simulink model "NTCM_Procedure"  (R2021a)
settings: Solver=FixedStepAuto  StartTime=0.0  StopTime=End_Time  FixedStep=Sample_Time  RelTol=1e-3  EnableMultiTasking=on
model workspace (MAT data in the model file):
  ErrCodeEl = Simulink.Parameter
  ErrCodeEl.Value = 1
  ErrCodeEl.DataType = 'uint16'
  ErrCodeEl.Dimensions = [1 1]
  ErrCodeIn = Simulink.Parameter
  ErrCodeIn.Value = 1
  ErrCodeIn.DataType = 'uint16'
  ErrCodeIn.Dimensions = [1 1]
  ErrCodeOut = Simulink.Parameter
  ErrCodeOut.Value = 1
  ErrCodeOut.DataType = 'uint16'
  ErrCodeOut.Dimensions = [1 1]
  ErrVarCheckIn = Simulink.Parameter
  ErrVarCheckIn.Value = [0; 0; 0; 0; 0; 0; 0; 0; 0; 0; 0; 0]
  ErrVarCheckIn.DataType = 'auto'
  ErrVarCheckIn.Dimensions = [12 1]
  ErrVarCheckOut = Simulink.Parameter
  ErrVarCheckOut.Value = [0; 0; 0]
  ErrVarCheckOut.DataType = 'auto'
  ErrVarCheckOut.Dimensions = [3 1]
  ErrVarEl = Simulink.Parameter
  ErrVarEl.Value = 0
  ErrVarEl.DataType = 'auto'
  ErrVarEl.Dimensions = [1 1]
  IPP_RefAltitude = Simulink.Parameter
  IPP_RefAltitude.Value = 450000
  IPP_RefAltitude.DataType = 'auto'
  IPP_RefAltitude.Dimensions = [1 1]
  LTd = Simulink.Parameter
  LTd.Value = 14
  LTd.DataType = 'auto'
  LTd.Dimensions = [1 1]
  NoErr = Simulink.Parameter
  NoErr.Value = 0
  NoErr.DataType = 'uint16'
  NoErr.Dimensions = [1 1]
  Pf1 = Simulink.Parameter
  Pf1.Value = 0.4
  Pf1.DataType = 'auto'
  Pf1.Dimensions = [1 1]
  RangeLwEl = Simulink.Parameter
  RangeLwEl.Value = 0
  RangeLwEl.DataType = 'auto'
  RangeLwEl.Dimensions = [1 1]
  RangeLwIn = Simulink.Parameter
  RangeLwIn.Value = [0; -4; -0.25; 1; 0; -90; -180; -4000; -90; -180; 450000; 0]
  RangeLwIn.DataType = 'auto'
  RangeLwIn.Dimensions = [12 1]
  RangeLwOut = Simulink.Parameter
  RangeLwOut.Value = [0; 0; 0]
  RangeLwOut.DataType = 'auto'
  RangeLwOut.Dimensions = [3 1]
  RangeUpEl = Simulink.Parameter
  RangeUpEl.Value = 1.57079632679
  RangeUpEl.DataType = 'auto'
  RangeUpEl.Dimensions = [1 1]
  RangeUpIn = Simulink.Parameter
  RangeUpIn.Value = [512; 4; 0.25; 366; 24; 90; 180; 400000; 90; 180; 600000000; 20000000000]
  RangeUpIn.DataType = 'auto'
  RangeUpIn.Dimensions = [12 1]
  RangeUpOut = Simulink.Parameter
  RangeUpOut.Value = [500; 1500; 1000000000000]
  RangeUpOut.DataType = 'auto'
  RangeUpOut.Dimensions = [3 1]
  Re = Simulink.Parameter
  Re.Value = 6371000
  Re.DataType = 'auto'
  Re.Dimensions = [1 1]
  doy_DAV = Simulink.Parameter
  doy_DAV.Value = 18
  doy_DAV.DataType = 'auto'
  doy_DAV.Dimensions = [1 1]
  doy_DSAV = Simulink.Parameter
  doy_DSAV.Value = 6
  doy_DSAV.DataType = 'auto'
  doy_DSAV.Dimensions = [1 1]
  k1 = Simulink.Parameter
  k1.Value = 0.92519
  k1.DataType = 'auto'
  k1.Dimensions = [1 1]
  k10 = Simulink.Parameter
  k10.Value = 1.20556
  k10.DataType = 'auto'
  k10.Dimensions = [1 1]
  k11 = Simulink.Parameter
  k11.Value = 1.41808
  k11.DataType = 'auto'
  k11.Dimensions = [1 1]
  k12 = Simulink.Parameter
  k12.Value = 0.13985
  k12.DataType = 'auto'
  k12.Dimensions = [1 1]
  k2 = Simulink.Parameter
  k2.Value = 0.16951
  k2.DataType = 'auto'
  k2.Dimensions = [1 1]
  k3 = Simulink.Parameter
  k3.Value = 0.00443
  k3.DataType = 'auto'
  k3.Dimensions = [1 1]
  k4 = Simulink.Parameter
  k4.Value = 0.06626
  k4.DataType = 'auto'
  k4.Dimensions = [1 1]
  k5 = Simulink.Parameter
  k5.Value = 0.00899
  k5.DataType = 'auto'
  k5.Dimensions = [1 1]
  k6 = Simulink.Parameter
  k6.Value = 0.21289
  k6.DataType = 'auto'
  k6.Dimensions = [1 1]
  k7 = Simulink.Parameter
  k7.Value = -0.15414
  k7.DataType = 'auto'
  k7.Dimensions = [1 1]
  k8 = Simulink.Parameter
  k8.Value = -0.38439
  k8.DataType = 'auto'
  k8.Dimensions = [1 1]
  k9 = Simulink.Parameter
  k9.Value = 1.14023
  k9.DataType = 'auto'
  k9.Dimensions = [1 1]
  lamGNP_deg = Simulink.Parameter
  lamGNP_deg.Value = -71.78
  lamGNP_deg.DataType = 'auto'
  lamGNP_deg.Dimensions = [1 1]
  phiGNP_deg = Simulink.Parameter
  phiGNP_deg.Value = 79.74
  phiGNP_deg.DataType = 'auto'
  phiGNP_deg.Dimensions = [1 1]
  phi_c1 = Simulink.Parameter
  phi_c1.Value = 16
  phi_c1.DataType = 'auto'
  phi_c1.Dimensions = [1 1]
  phi_c2 = Simulink.Parameter
  phi_c2.Value = -10
  phi_c2.DataType = 'auto'
  phi_c2.Dimensions = [1 1]
  sigma_c1 = Simulink.Parameter
  sigma_c1.Value = 12
  sigma_c1.DataType = 'auto'
  sigma_c1.Dimensions = [1 1]
  sigma_c2 = Simulink.Parameter
  sigma_c2.Value = 13
  sigma_c2.DataType = 'auto'
  sigma_c2.Dimensions = [1 1]
Description:
  | Model NTCM Procedure
settings Model: ModifiedByFormat=Francesco Menzione  OrderedModelArguments=off  Creator=Francesco Menzione  LastModifiedBy=Francesco Menzione
settings DataIOCC: ReturnWorkspaceOutputs=off  SignalLoggingName=logsout_new
settings OptimizationCC: UseDivisionForNetSlopeComputation=on  UseFloatMulNetSlope=on  UseSpecifiedMinMax=on  BufferReuse=off  PassReuseOutputArgsAs=Individual arguments  ZeroExternalMemoryAtStartup=off  ZeroInternalMemoryAtStartup=off  EfficientFloat2IntCast=on  LifeSpan=2  EfficientTunableParamExpr=on
settings DebuggingCC: ParameterTunabilityLossMsg=error  AssertControl=DisableAll  SFMachineParentedDataDiag=warning
settings HardwareCC: ProdBitPerPointer=32  ProdBitPerSizeT=32  ProdBitPerPtrDiffT=32  ProdLargestAtomicInteger=LongLong  ProdLargestAtomicFloat=Double  ProdEndianess=BigEndian  ProdWordSize=32  ProdLongLongMode=on  ProdHWDeviceType=Custom Processor->Custom
settings SFSimCC: MATLABDynamicMemAlloc=off
settings RTWCC: SystemTargetFile=ert.tlc  TemplateMakefile=ert_default_tmf  GenerateReport=on  CustomDefine=CheckOn=1  Toolchain=MinGW64 | gmake (64-bit Windows)  BuildConfiguration=Faster Runs  LaunchReport=on  PortableWordSizes=on  CodeExecutionProfiling=on  CodeProfilingInstrumentation=detailed  GenerateTraceReportSl=on  GenerateTraceReportSf=on  GenerateTraceReportEml=on  GenerateWebview=on  GenerateCodeMetricsReport=on  CheckMdlBeforeBuild=Warning
settings CodeAppCC: IgnoreCustomStorageClasses=off  OperatorAnnotations=on  SimulinkDataObjDesc=on  CustomSymbolStrFcn=$M$F  CustomSymbolStrFcnArg=$N$M  CustomSymbolStrBlkIO=lOut_$N$M  InsertBlockDesc=on  SimulinkBlockComments=off
settings ERTTargetCC: TargetLangStandard=C99 (ISO)  UtilityFuncGeneration=Shared location  GenerateSampleERTMain=on  CombineSignalStateStructs=on  SuppressErrorStatus=on  CodeInterfacePackaging=Reusable function  SupportNonFinite=off  SupportComplex=off  RemoveResetFunc=off  ParenthesesLevel=Maximum  CastingMode=Standards  RootIOFormat=Structure reference  ERTSrcFileBannerTemplate=JRCert_code_template.cgt  ERTHdrFileBannerTemplate=JRCert_code_template.cgt  ERTDataSrcFileTemplate=JRCert_code_template.cgt  ERTDataHdrFileTemplate=JRCert_code_template.cgt  ERTCustomFileTemplate=example_file_process.tlc  EnableSignedLeftShifts=off  EnableSignedRightShifts=off

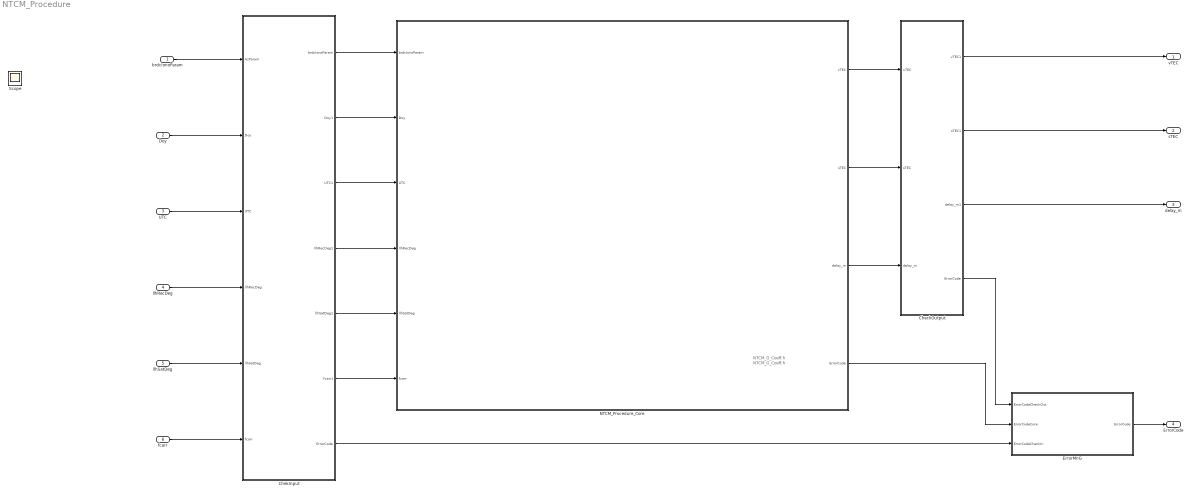
== system NTCM_Procedure ==
  note: NTCM_G_Coeff.h
  note: NTCM_G_Coeff.h
  brdcIonoParam : Inport  PortDimensions=[3,1]
  Doy : Inport  Port=2  PortDimensions=1
  UTC : Inport  Port=3  PortDimensions=1
  llhRecDeg : Inport  Description=dxdxxdxhx  Port=4  PortDimensions=[3,1]
  llhSatDeg : Inport  Port=5  PortDimensions=[3,1]
  fcarr : Inport  Port=6  PortDimensions=1
  CheckOutput : Subsystem  Description=|  TreatAsAtomicUnit=on  RTWFcnName=CheckOutput
      | FUNCTION:
      |    ------
      |    The function check that all output lie within the expected range and perform
      |    correspondent saturation when needed
      |    
      |    INPUT:
      |    ------
      | /n vTEC => Vertical TEC [TECU]
      | /n sTEC => Slant TEC [TECU]
      | /n delay_m=> Ionospheric Delay [m]
      | /n llhRecDeg => User position in Longitude[rad], Latitude[rad], height[m] 
      | /n llhSatDeg => Satellite position in Longitude[rad], Latitude[rad], height[m]  
      | /n fcarr => Carrier frequency
      |    
      |    OUTPUT:
      |    ------
      | /n lOutCheck_Input => Validated  Output vector [1,2,3]
      | /n lOut_ErrorCheckIn =>Validity  Output flag [1,2,3]
      settings: RTWFcnNameOpts=User specified  RTWFileNameOpts=Use function name
  ChekInput : Subsystem  Description=|  TreatAsAtomicUnit=on  RTWFcnName=ChekInput
      | FUNCTION:
      |    ------
      |    The function check that all input lie within the expected range and perform
      |    correspondent saturation when needed
      |    
      |    INPUT:
      |    ------
      |    AzPara => Az0, Az1 and Az2 Iono Parameters broadcasted by Galileo
      | \n Doy => Day of the year 
      | \n UTC => UTC Time in hours (0 for midnight)
      | \n llhRecDeg => User position in Longitude[rad], Latitude[rad], height[m] 
      | \n llhSatDeg => Satellite position in Longitude[rad], Latitude[rad], height[m]  
      | \n fcarr => Carrier frequency
      |    
      |    OUTPUT:
      | -  -----
      |    lOutCheck_Input => Validated Input vector [1,...12]
      | \n lOut_ErrorCheckIn =>Validity Flags [1,...12]
      settings: RTWFcnNameOpts=User specified  RTWFileNameOpts=Use function name
  ErrorMnG : Subsystem  Description=|  TreatAsAtomicUnit=on  RTWFcnName=ErrorMnG
      | ChekOutput
      |    FUNCTION:
      |    ------
      |    The function ccollect all errors log in a unique vector of unsigned integers
      |    
      |    INPUT:
      |    ------
      |    ErrorCodeCheckOut => Error Code for Output Interface 
      | /n ErrorCodeCore => Error Code for Core 
      | /n ErrorCodeCheckIn =>Error Code for Input  Interface 
      |    
      |    OUTPUT:
      |    ------
      | /n ErrorCode =>Final Err Code Vector [ ErrorCodeCheckOut,ErrorCodeCore,ErrorCodeCheckIn
      settings: RTWFcnNameOpts=User specified  RTWFileNameOpts=Use function name
  NTCM_Procedure_Core : Subsystem  Description=|  TreatAsAtomicUnit=on  RTWFcnName=NTCM_Procedure_Core
      | <strong> FUNCTION </strong>
      |     The core function implements the step-by-step procedure as described in [1].
      |    The "core" suffix aim at sparating this pure algorithmic block from any consistency/control
      |    or I/O logic implemented externally by the user ( the check-in/checkout steps included in the
      |    overall procedure are provided just an example of possible wrapping. It is worthy to remind
      |    that in order to implement the ionospheric algorithm for Galileo single frequency receivers
      |    for each satellite-user line-of-sight the following steps shall be followed:
      |    \n 1) Obtain estimates of user receiver position (lat,long,h)_i, satellite position (lat,long,h)_j
      |    \n 2) Universal Time (UT), in terms of time of day and month
      |    \n 3) Obtain Effective Ionisation Level Azpar and broadcast coefficients (a_i0,a_i1,a_i2 )
      |    \n 4)Calculate satellite elevation (E) and azimuth (A) angles
      |    \n 5)Calculate ionospheric pierce point location for the user-to-satellite
      |    \n 6) Call NTCM_G to calculate VTEC at pierce point location and local time (LT)
      |    \n   (Section 2.5.4 in[1] provides a formula to convert UT to LT).
      |    \n 7) Calculate ionospheric Mapping Function (MF) using the equation provided in Section 2.5.8.
      |    \n 8) Convert VTEC to STEC using the ionospheric mapping function.
      |    \n 9) Convert STEC to time delay using Eq. 1 in[1] for the corresponding frequency to obtain
      |    \n the correction
      |    \n 10) Apply correction to selected link
      | 
      |    @param[in] AzPara  		=> alpha0, alpha1, and alpha2 Iono Parameters broadcasted by Galileo
      |    @param[in] Doy  		=> Day of the year
      |    @param[in] UTC   		=> UTC Time in hours (0 for midnight)
      |    @param[in] llhRecDeg   		=> User position in Longitude[rad], Latitude[rad], height[m]
      |    @param[in] llhSatDeg  		=> Satellite position in Longitude[rad], Latitude[rad], height[m]
      |    @param[in] fcarr  		=> Carrier frequency
      | 
      |    @param[out] vTEC  		=> Vertical TEC
      |    @param[out] sTEC  		=> Slant TEC
      |    @param[out] delay_m  		=> Signal propagation time delay in [m]
      |    @param[out] ErrorCode  		=> Error Code (optional)
      | 
      |  
      |  <strong> Tuning Constant </strong>
      |   <table>
      |  <tr><th> Label                      <th>Value       
      |  <tr><td> ErrCodeEl <td> 2U 
      |  <tr><td> ErrCodeEl  		<td>2U                        
      |  <tr><td> ErrCodeIn  		<td>1U
      |  <tr><td> ErrCodeOut  	<td>3U
      |  <tr><td> IPP_RefAltitude <td> 450000.0                  
      |  <tr><td> LTd  			<td>14.0
      |  <tr><td> NoErr  			<td>0U
      |  <tr><td> Pf1  			<td>0.4
      |  <tr><td> doy_DAV  		<td>18.0
      |  <tr><td> doy_DSAV  		<td>6.0
      |  <tr><td> lamGNP_deg  	<td>-71.78
      |  <tr><td> phiGNP_deg  	<td>79.74
      |  <tr><td> phi_c1  		<td>16.0
      |  <tr><td> phi_c2  		<td>-10.0
      |  <tr><td> sigma_c1  		<td>12.0
      |  <tr><td> sigma_c2  		<td>13.0
      |  <tr><td> k1  			<td>0.92519
      |  <tr><td> k10  			<td>1.20556
      |  <tr><td> k11  			<td>1.41808
      |  <tr><td> k12  			<td>0.13985
      |  <tr><td> k2  			<td>0.16951
      |  <tr><td> k3  			<td>0.00443
      |  <tr><td> k4  			<td>0.06626
      |  <tr><td> k5  			<td>0.00899
      |  <tr><td> k6  			<td>0.21289
      |  <tr><td> k7  			<td>-0.15414
      |  <tr><td> k8  			<td>-0.38439
      |  <tr><td> k9  			<td>1.14023
      | </table>
      | @ingroup NTCM_Procedure
      | @file
      settings: RTWFcnNameOpts=User specified  RTWFileNameOpts=Use function name
  vTEC : Outport
  sTEC : Outport  Port=2
  delay_m : Outport  Port=3
  ErrorCode : Outport  Port=4
  Scope : Scope
  wires:
  CheckOutput/1(vTEC1) -> vTEC/1
  CheckOutput/2(sTEC1) -> sTEC/1
  ErrorMnG/1(ErrorCode) -> ErrorCode/1
  CheckOutput/3(delay_m1) -> delay_m/1
  brdcIonoParam/1 -> ChekInput/1(AzParam)
  Doy/1 -> ChekInput/2(Doy)
  UTC/1 -> ChekInput/3(UTC)
  llhRecDeg/1 -> ChekInput/4(llhRecDeg)
  llhSatDeg/1 -> ChekInput/5(llhSatDeg)
  fcarr/1 -> ChekInput/6(fcarr)
  ChekInput/1(brdcIonoParam) -> NTCM_Procedure_Core/1(brdcIonoParam)
  ChekInput/2(Doy1) -> NTCM_Procedure_Core/2(Doy)
  ChekInput/3(UTC1) -> NTCM_Procedure_Core/3(UTC)
  ChekInput/4(llhRecDeg1) -> NTCM_Procedure_Core/4(llhRecDeg)
  ChekInput/5(llhSatDeg1) -> NTCM_Procedure_Core/5(llhSatDeg)
  ChekInput/6(fcarr1) -> NTCM_Procedure_Core/6(fcarr)
  NTCM_Procedure_Core/1(vTEC) -> CheckOutput/1(vTEC)
  NTCM_Procedure_Core/2(sTEC) -> CheckOutput/2(sTEC)
  NTCM_Procedure_Core/3(delay_m) -> CheckOutput/3(delay_m)
  CheckOutput/4(ErrorCode) -> ErrorMnG/1(ErrorCodeCheckOut)
  NTCM_Procedure_Core/4(ErrorCode) -> ErrorMnG/2(ErrorCodeCore)
  ChekInput/7(ErrorCode) -> ErrorMnG/3(ErrorCodeCheckIn)

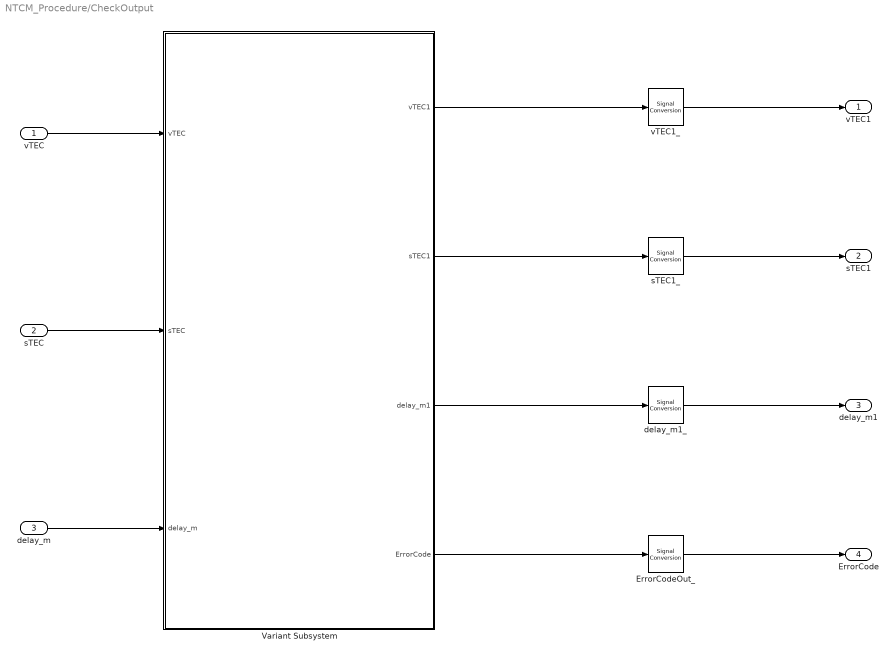
== system NTCM_Procedure/CheckOutput ==
  vTEC : Inport
  sTEC : Inport  Port=2
  delay_m : Inport  Port=3
  ErrorCodeOut_ : SignalConversion  OverrideOpt=off
  Variant Subsystem : Subsystem  Variant=on  VariantActivationTime=code compile
  delay_m1_ : SignalConversion  OverrideOpt=off
  sTEC1_ : SignalConversion  OverrideOpt=off
  vTEC1_ : SignalConversion  OverrideOpt=off
  vTEC1 : Outport
  sTEC1 : Outport  Port=2
  delay_m1 : Outport  Port=3
  ErrorCode : Outport  Port=4
  wires:
  Variant Subsystem/2(sTEC1) -> sTEC1_/1
  delay_m/1 -> Variant Subsystem/3(delay_m)
  vTEC/1 -> Variant Subsystem/1(vTEC)
  Variant Subsystem/1(vTEC1) -> vTEC1_/1
  Variant Subsystem/3(delay_m1) -> delay_m1_/1
  Variant Subsystem/4(ErrorCode) -> ErrorCodeOut_/1
  sTEC/1 -> Variant Subsystem/2(sTEC)
  vTEC1_/1 -> vTEC1/1
  sTEC1_/1 -> sTEC1/1
  delay_m1_/1 -> delay_m1/1
  ErrorCodeOut_/1 -> ErrorCode/1

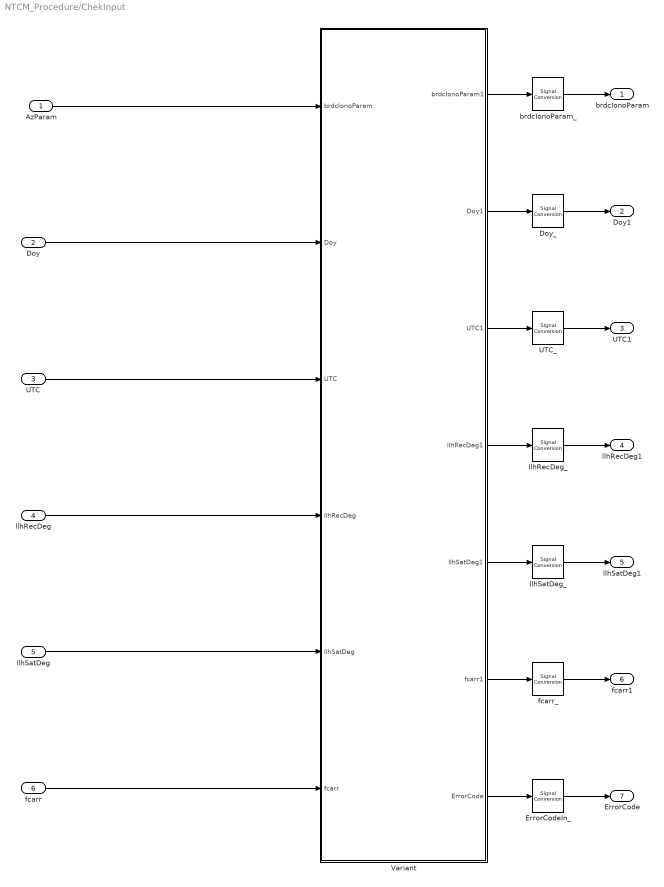
== system NTCM_Procedure/ChekInput ==
  AzParam : Inport
  Doy : Inport  Port=2
  UTC : Inport  Port=3
  llhRecDeg : Inport  Port=4
  llhSatDeg : Inport  Port=5
  fcarr : Inport  Port=6
  Doy_ : SignalConversion  OverrideOpt=off
  ErrorCodeIn_ : SignalConversion  OverrideOpt=off
  UTC_ : SignalConversion  OverrideOpt=off
  Variant : Subsystem  Variant=on  VariantActivationTime=code compile
  brdcIonoParam_ : SignalConversion  OverrideOpt=off
  fcarr_ : SignalConversion  OverrideOpt=off
  llhRecDeg_ : SignalConversion  OverrideOpt=off
  llhSatDeg_ : SignalConversion  OverrideOpt=off
  brdcIonoParam : Outport
  Doy1 : Outport  Port=2
  UTC1 : Outport  Port=3
  llhRecDeg1 : Outport  Port=4
  llhSatDeg1 : Outport  Port=5
  fcarr1 : Outport  Port=6
  ErrorCode : Outport  Port=7
  wires:
  fcarr/1 -> Variant/6(fcarr)
  Variant/1(brdcIonoParam1) -> brdcIonoParam_/1
  Variant/2(Doy1) -> Doy_/1
  Variant/4(llhRecDeg1) -> llhRecDeg_/1
  Variant/7(ErrorCode) -> ErrorCodeIn_/1
  Variant/6(fcarr1) -> fcarr_/1
  Variant/3(UTC1) -> UTC_/1
  Variant/5(llhSatDeg1) -> llhSatDeg_/1
  UTC/1 -> Variant/3(UTC)
  AzParam/1 -> Variant/1(brdcIonoParam)
  llhRecDeg/1 -> Variant/4(llhRecDeg)
  llhSatDeg/1 -> Variant/5(llhSatDeg)
  Doy/1 -> Variant/2(Doy)
  brdcIonoParam_/1 -> brdcIonoParam/1
  Doy_/1 -> Doy1/1
  UTC_/1 -> UTC1/1
  llhRecDeg_/1 -> llhRecDeg1/1
  llhSatDeg_/1 -> llhSatDeg1/1
  fcarr_/1 -> fcarr1/1
  ErrorCodeIn_/1 -> ErrorCode/1

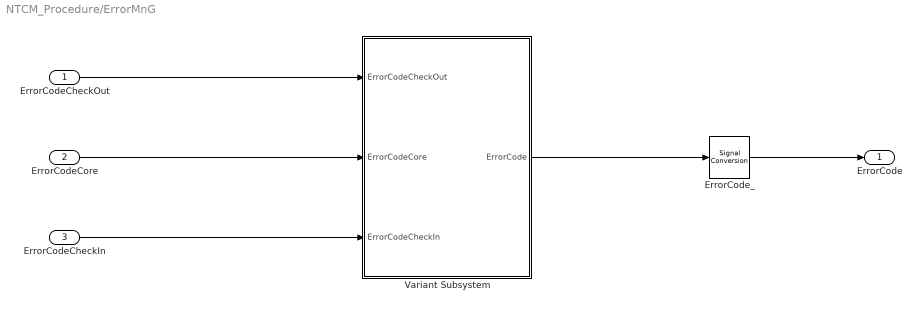
== system NTCM_Procedure/ErrorMnG ==
  ErrorCodeCheckOut : Inport
  ErrorCodeCore : Inport  Port=2
  ErrorCodeCheckIn : Inport  Port=3
  ErrorCode_ : SignalConversion  OverrideOpt=off
  Variant Subsystem : Subsystem  Variant=on  VariantActivationTime=code compile
  ErrorCode : Outport
  wires:
  Variant Subsystem/1(ErrorCode) -> ErrorCode_/1
  ErrorCodeCheckOut/1 -> Variant Subsystem/1(ErrorCodeCheckOut)
  ErrorCodeCore/1 -> Variant Subsystem/2(ErrorCodeCore)
  ErrorCodeCheckIn/1 -> Variant Subsystem/3(ErrorCodeCheckIn)
  ErrorCode_/1 -> ErrorCode/1

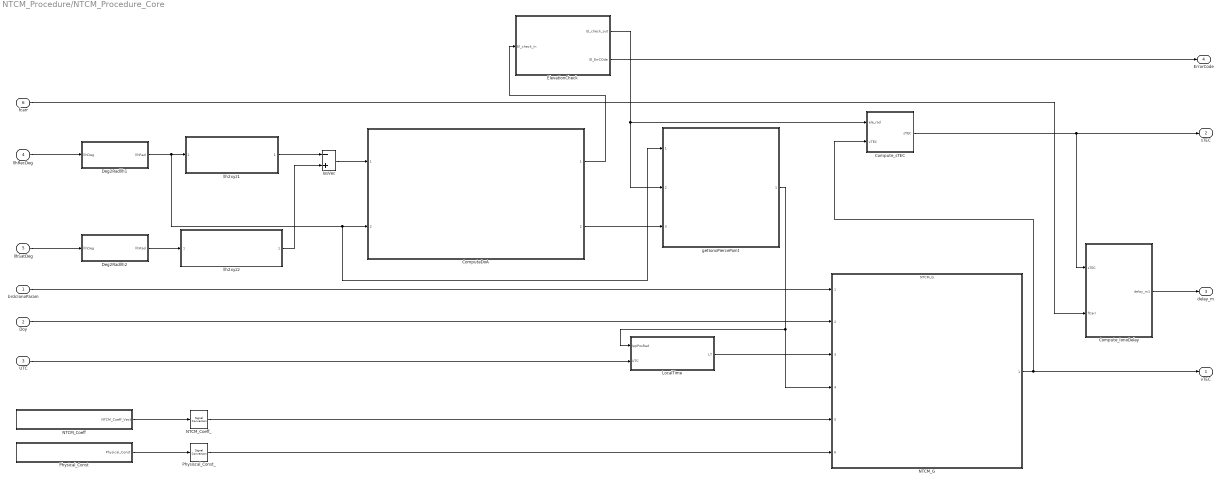
== system NTCM_Procedure/NTCM_Procedure_Core ==
  brdcIonoParam : Inport  PortDimensions=[3,1]
  Doy : Inport  Port=2  PortDimensions=1
  UTC : Inport  Port=3
  llhRecDeg : Inport  Port=4  PortDimensions=[3,1]
  llhSatDeg : Inport  Port=5  PortDimensions=[3,1]
  fcarr : Inport  Port=6
  ComputeDoA : Subsystem  Description=|  TreatAsAtomicUnit=on  RTWFcnName=ComputeDoA  ReferencedSubsystem=ComputeDoA
      | @ingroup NTCM_Procedure
      |    <strong> FUNCTION </strong>
      | 
      |    This module computes the satellite azimuth and elevation angles (Described in Section 2.5.2)
      |    
      |    @param[in] losVec 		=> Line of sight vector
      |    @param[in] llhUserRad 		=>  Receiver position Latitude [rad], Longitude[rad], height[m]
      | 
      |    @param[out] SvDoAEleRad 		=>  Line of sight Elevation
      |    @param[out] SvDoAAzRad  		=>  Line of sight Azimuth
      | 
      | @file
      settings: RTWFcnNameOpts=User specified  RTWFileNameOpts=Use function name
  Compute_IonoDelay : Subsystem  Description=|  TreatAsAtomicUnit=on  RTWFcnName=Compute_IonoDelay
      | @ingroup NTCM_Procedure
      | 
      |    <strong> FUNCTION </strong>
      |    Compute ionospheric Delay
      | 
      |    @param[in] sTEC		=> Slant TEC
      |    @param[in] fCarr		=> Carrier Frequency
      |    @param[out] delay_m		=>ionospheric Delay[m] 
      | 
      | @file
      settings: RTWFcnNameOpts=User specified  RTWFileNameOpts=Use function name
  Compute_sTEC : Subsystem  Description=|  TreatAsAtomicUnit=on  RTWFcnName=Compute_sTEC
      | @ingroup NTCM_Procedure
      | 
      |    <strong> FUNCTION </strong>
      |    This module computes the Mapping Function and converts the estimated VTEC to STEC (Described in Section 2.5.8).
      |    
      |    @param[in] ele_rad 		=> Satellite elevation
      |    @param[in] vTEC 		=>  Vertical Total Electron Content [TECU]
      | 
      |    @param[out] sTEC 		=>  Slant Total Electron Content [TECU]
      | 
      | @file
      settings: RTWFcnNameOpts=User specified  RTWFileNameOpts=Use function name
  Deg2Radllh1 : MATLAB Function  TreatAsAtomicUnit=on  RTWFcnName=llh2xyz
      settings: RTWSystemCode=Inline  RTWFileNameOpts=Use function name
  Deg2Radllh2 : MATLAB Function  TreatAsAtomicUnit=on  RTWFcnName=llh2xyz
      settings: RTWSystemCode=Inline  RTWFileNameOpts=Use function name
  ElevationCheck : Subsystem  Description=|  TreatAsAtomicUnit=on  RTWFcnName=ElevetionCheck
      | <strong> FUNCTION </strong>
      |    Positivity elevetaion check 
      |    
      |    @param[in] El_check_in/t/t Satellite Elevation [rad]
      |    
      |    @param[out] El_check_out/t/t Limited Elevation 
      |    @param[out] El_ErrCOde /t/t Elevation out of range error code
      settings: RTWFcnNameOpts=User specified  RTWFileNameOpts=Use function name
  LocalTime : Subsystem  Description=|  TreatAsAtomicUnit=on  RTWFcnName=ComputeLocalTime
      | @ingroup NTCM_Procedure
      |    FUNCTION:
      |    ------
      |    This module computes the local time LT given the pierce point longitude and UT. 
      |    
      |    @param[in] IppPosRad 		=> Pierce Point Position in  Latitude[rad], Longitude[rad], height[m]
      |    @param[in] UTC		=> utc time
      |    @param[out] LT		=> Local Time
      | 
      | @file
      settings: RTWFcnNameOpts=User specified  RTWFileNameOpts=Use function name
  NTCM_Coeff : Subsystem  RTWFcnName=NTCM_Coeff
      settings: RTWSystemCode=Inline  RTWFcnNameOpts=User specified  FunctionInterfaceSpec=Allow arguments (Optimized)
  NTCM_Coeff_ : SignalConversion  Description=Allocate NTCM Coeff as Input Vector  OverrideOpt=on
  NTCM_G : ModelReference  Description=|  ModelNameDialog=NTCM_G.slx  SimulationMode=Normal  ModelReferenceVersion=1.0
      | <strong> FUNCTION </strong>
      |    The NTCM G is an empirical model that allows easy determination of global TEC.
      |    The model describes the main ionospheric features with good quality using a small
      |    number of model coefficients and parameters. The non-linear approach needs only 12
      |    coefficients and a few empirically fixed parameters for describing the broad spectrum
      |    of TEC variation for all levels of solar activity
      |    
      |    @param[in] brdcIonoParam		=> ai0,ai1,ai2 Effective Ionisation Level parameters broadcast in the Galileo Navigation Message
      |    @param[in] doy 		=> Day of the Year
      |    @param[in] LT 		=> Local Time [hours]
      |    @param[in] IppCoord 		=> Pierce Point Coordinates in  Latitude[rad], Longitude[rad]
      |    @param[in] NTCM_Coeff_Vect 		=> NTCM model coefficients k1,k2,..,k12 (Described in Section 2.4.3)
      |    @param[in] NTCM_Phys_Cons 		=> Vector of Pysical Constant 
      |    
      |    @param[out] vTEC_0 		=> Total Electron Content [TECU]
      | 
      | @ingroup NTCM_Procedure
      | @ingroup NTCM_G
      | @file
  Physical_Const : Subsystem  RTWFcnName=Physiscal_Const
      settings: RTWFcnNameOpts=User specified  FunctionInterfaceSpec=Allow arguments (Optimized)
  Physiscal_Const_ : SignalConversion  Description=Allocate NTCM Physiscal Const as Input Vector  OverrideOpt=on
  getIonoPiercePoint : Subsystem  Description=|  TreatAsAtomicUnit=on  RTWFcnName=getIonoPiercePoint  ReferencedSubsystem=getIonoPiercePoint
      | @ingroup NTCM_Procedure   
      | 
      | <strong> FUNCTION </strong>
      |    This module computes the geographic latitude and longitude of the Ionospheric Pierce Point (IPP) (Described in Section 2.5.2).
      |    IPP is the point where the Line of Sight (LoS) intersects the reference ionospheric layer, this latter set at an altitude of 450Km.
      | 
      |    @param[in] llhUser 		=> Receiver position in  Latitude[rad], Longitude[rad], height[m]
      |    @param[in] ElRad 		=> Elevation (DoA) [rad]
      |    @param[in] AzRad 		=> Azimuth (DoA) [rad]
      |    
      |    @param [out] IppCoord 		=>Pierce Point coordinates in  Latitude[rad], Longitude[rad]
      | 
      | @file
      settings: RTWFcnNameOpts=User specified  RTWFileNameOpts=Use function name
  llh2xyz1 : Subsystem  Description=|  TreatAsAtomicUnit=on  RTWFcnName=llh2xyz_Rec  ReferencedSubsystem=llh2xyz
      | @ingroup NTCM_Procedure
      |    
      |    <strong> FUNCTION </strong>
      |    This module converts the receiver geodetic WGS84 coordinates to ECEF (Described in Sec.2.5.1)
      |       
      |    @param[in] llh 		=> WGS84 coordinates in Latitude[rad], Longitude[rad], height[m]
      |    @param[out] xyz 		=> ECEF coordinates in x[m], y[m], z[m]
      |    
      |    @file
      settings: RTWFcnNameOpts=User specified  RTWFileNameOpts=Use function name
  llh2xyz2 : Subsystem  Description=|  TreatAsAtomicUnit=on  RTWFcnName=llh2xyz_Sat  ReferencedSubsystem=llh2xyz
      | @ingroup NTCM_Procedure 
      | 
      |    <strong> FUNCTION </strong>
      |    This module converts the SV geodetic WGS84 coordinates to ECEF (Described in Sec.2.5.1)
      |    @param[in] llh 		=> WGS84 coordinates in Latitude[rad], Longitude[rad], height[m]
      |    @param[out] xyz 		=> ECEF coordinates in x[m], y[m], z[m]
      |    
      |    @file
      settings: RTWFcnNameOpts=User specified  RTWFileNameOpts=Use function name
  losVec : Sum  Inputs=-+
  vTEC : Outport
  sTEC : Outport  Port=2
  delay_m : Outport  Port=3
  ErrorCode : Outport  Port=4
  wires:
  Deg2Radllh1/1(llhRad) -> getIonoPiercePoint/1, ComputeDoA/2, llh2xyz1/1
  getIonoPiercePoint/1 -> NTCM_G/4, LocalTime/1(IppPosRad)
  NTCM_Coeff/1(NTCM_Coeff_Vect) -> NTCM_Coeff_/1
  losVec/1 -> ComputeDoA/1
  llh2xyz1/1 -> losVec/1
  Doy/1 -> NTCM_G/2
  llhSatDeg/1 -> Deg2Radllh2/1(llhDeg)
  Physical_Const/1(Physical_Const) -> Physiscal_Const_/1
  llh2xyz2/1 -> losVec/2
  brdcIonoParam/1 -> NTCM_G/1
  Deg2Radllh2/1(llhRad) -> llh2xyz2/1
  ComputeDoA/2 -> getIonoPiercePoint/3
  llhRecDeg/1 -> Deg2Radllh1/1(llhDeg)
  Compute_IonoDelay/1(delay_m1) -> delay_m/1
  NTCM_G/1 -> vTEC/1, Compute_sTEC/2(vTEC)
  Compute_sTEC/1(sTEC) -> Compute_IonoDelay/1(sTEC), sTEC/1
  fcarr/1 -> Compute_IonoDelay/2(fCarr)
  UTC/1 -> LocalTime/2(UTC)
  LocalTime/1(LT) -> NTCM_G/3
  ElevationCheck/1(El_check_out) -> getIonoPiercePoint/2, Compute_sTEC/1(ele_rad)
  ElevationCheck/2(El_ErrCOde) -> ErrorCode/1
  ComputeDoA/1 -> ElevationCheck/1(El_check_in)
  NTCM_Coeff_/1 -> NTCM_G/5
  Physiscal_Const_/1 -> NTCM_G/6

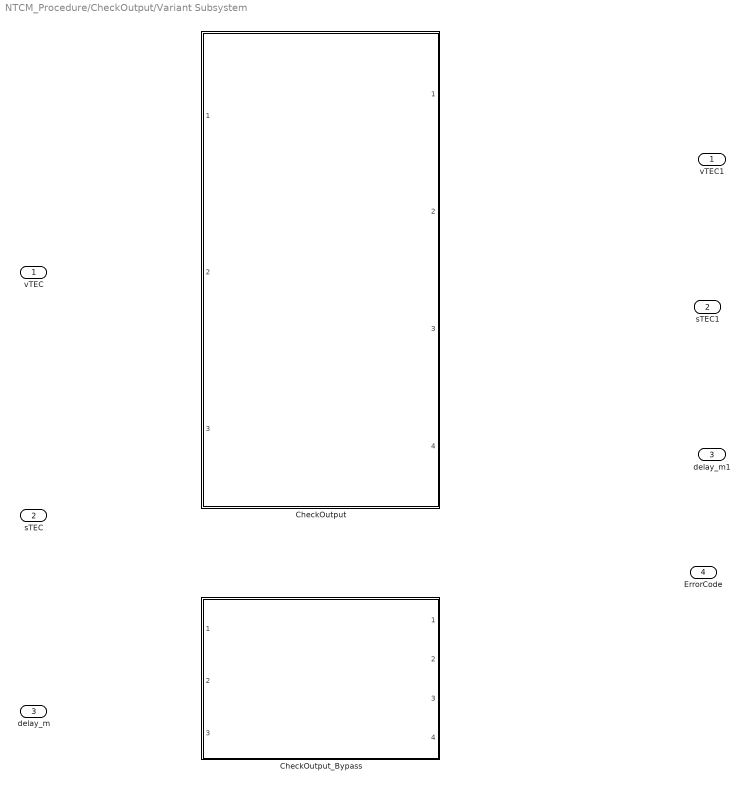
== system NTCM_Procedure/CheckOutput/Variant Subsystem ==
  vTEC : Inport
  sTEC : Inport  Port=2
  delay_m : Inport  Port=3
  CheckOutput : Subsystem  Description=|  TreatAsAtomicUnit=on  RTWFcnName=CheckOutput  VariantControl=CheckFlag  ReferencedSubsystem=CheckOutput
      | ChekIn
      |  FUNCTION:
      |  ------
      |  The function check that all output lie within the expected range and perform
      |  correspondent saturation when needed
      | 
      |  INPUT:
      |  ------
      |  vTEC => Vertical TEC [TECU]
      |  sTEC => Slant TEC [TECU]
      |  delay_m=> Ionospheric Delay [m]
      |  llhRecDeg => User position in Longitude[rad], Latitude[rad], height[m] 
      |  llhSatDeg => Satellite position in Longitude[rad], Latitude[rad], height[m]  
      |  fcarr => Carrier frequency
      | 
      |  OUTPUT:
      | ------
      |  lOutCheck_Input => Validated  Output vector [1,2,3]
      |  lOut_ErrorCheckIn =>Validity  Output flag [1,...12]
      settings: RTWFcnNameOpts=User specified  RTWFileNameOpts=Use function name
  CheckOutput_Bypass : Subsystem  TreatAsAtomicUnit=on  VariantControl=(default)  ReferencedSubsystem=CheckOutput_Bypass
  vTEC1 : Outport
  sTEC1 : Outport  Port=2
  delay_m1 : Outport  Port=3
  ErrorCode : Outport  Port=4

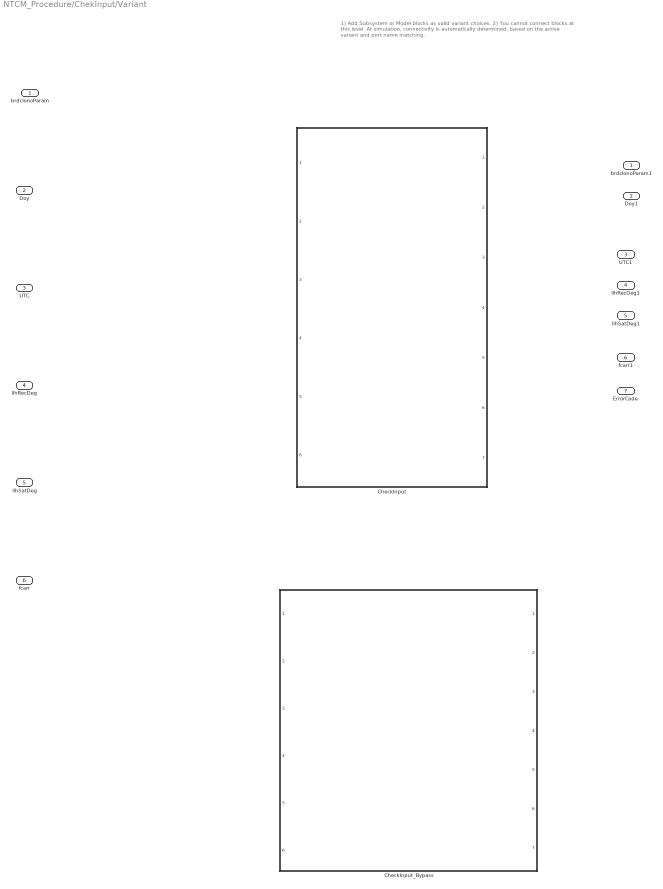
== system NTCM_Procedure/ChekInput/Variant ==
  note: 1) Add Subsystem or Model blocks as valid variant choices.
      | 2) You cannot connect blocks at this level. At simulation, connectivity is automatically
      | determined, based on the active variant and port name matching.
  brdcIonoParam : Inport  PortDimensions=[3,1]
  Doy : Inport  Port=2  PortDimensions=1
  UTC : Inport  Port=3  PortDimensions=1
  llhRecDeg : Inport  Description=dxdxxdxhx  Port=4  PortDimensions=[3,1]
  llhSatDeg : Inport  Port=5  PortDimensions=[3,1]
  fcarr : Inport  Port=6  PortDimensions=1
  CheckInput : Subsystem  Description=|  TreatAsAtomicUnit=on  RTWFcnName=CheckInput  VariantControl=CheckFlag  ReferencedSubsystem=CheckInput
      | ChekInput
      |  FUNCTION:
      |  ------
      |  The function check that all input lie within the expected range and perform
      |  correspondent saturation when needed
      | 
      |  INPUT:
      |  ------
      |  AzPara => Az0, Az1 and Az2 Iono Parameters broadcasted by Galileo
      |  Doy => Day of the year 
      |  UTC => UTC Time in hours (0 for midnight)
      |  llhRecDeg => User position in Longitude[rad], Latitude[rad], height[m] 
      |  llhSatDeg => Satellite position in Longitude[rad], Latitude[rad], height[m]  
      |  fcarr => Carrier frequency
      | 
      |  OUTPUT:
      | ------
      |  lOutCheck_Input => Validated Input vector [1,...12]
      |  lOut_ErrorCheckIn =>Validity Flags [1,...12]
      settings: RTWFcnNameOpts=User specified  RTWFileNameOpts=Use function name
  CheckInput_Bypass : Subsystem  TreatAsAtomicUnit=on  VariantControl=(default)  ReferencedSubsystem=CheckInput_Bypass
  brdcIonoParam1 : Outport
  Doy1 : Outport  Port=2
  UTC1 : Outport  Port=3
  llhRecDeg1 : Outport  Port=4
  llhSatDeg1 : Outport  Port=5
  fcarr1 : Outport  Port=6
  ErrorCode : Outport  Port=7

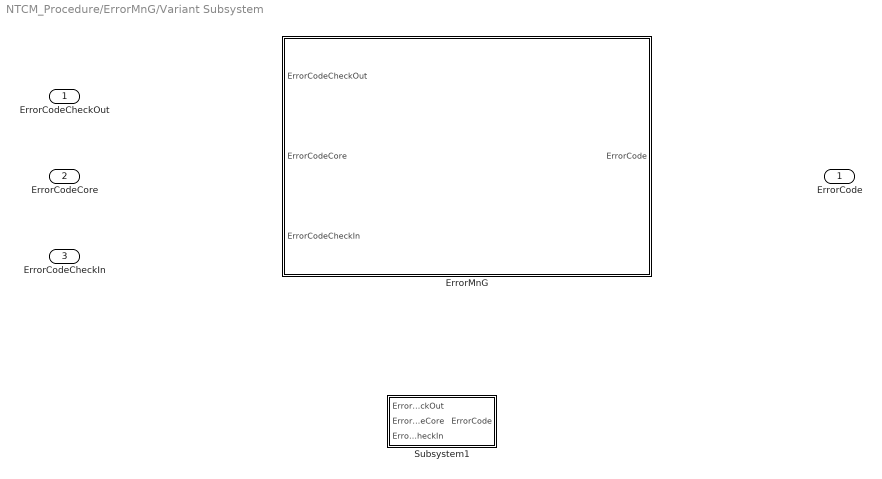
== system NTCM_Procedure/ErrorMnG/Variant Subsystem ==
  ErrorCodeCheckOut : Inport
  ErrorCodeCore : Inport  Port=2
  ErrorCodeCheckIn : Inport  Port=3
  "ErrorMnG " : Subsystem  TreatAsAtomicUnit=on  RTWFcnName=ErrorMng  VariantControl=CheckFlag
      settings: RTWFcnNameOpts=User specified  RTWFileNameOpts=Use function name
  Subsystem1 : Subsystem  TreatAsAtomicUnit=on  VariantControl=(default)
  ErrorCode : Outport

== system NTCM_Procedure/NTCM_Procedure_Core/Compute_IonoDelay ==
  sTEC : Inport
  fCarr : Inport  Port=2
  Compute_Delay : MATLAB Function  RTWFcnName=Compute_Delay
      settings: RTWFileNameOpts=Use function name  FunctionInterfaceSpec=Allow arguments (Optimized)
  delay_m1_ : SignalConversion  OverrideOpt=off
  delay_m1 : Outport
  wires:
  fCarr/1 -> Compute_Delay/2(fCarr)
  Compute_Delay/1(delay_m) -> delay_m1_/1
  sTEC/1 -> Compute_Delay/1(sTEC)
  delay_m1_/1 -> delay_m1/1

== system NTCM_Procedure/NTCM_Procedure_Core/Compute_sTEC ==
  ele_rad : Inport
  vTEC : Inport  Port=2
  Mapping_fun : MATLAB Function  RTWFcnName=Mapping_fun
      settings: AttributesFormatString=%<Abstract>  RTWFileNameOpts=Use function name  FunctionInterfaceSpec=Allow arguments (Optimized)
  sTEC_ : SignalConversion  OverrideOpt=off
  sTEC : Outport
  wires:
  vTEC/1 -> Mapping_fun/1(vTEC)
  Mapping_fun/1(sTEC) -> sTEC_/1
  ele_rad/1 -> Mapping_fun/2(ele_rad)
  sTEC_/1 -> sTEC/1

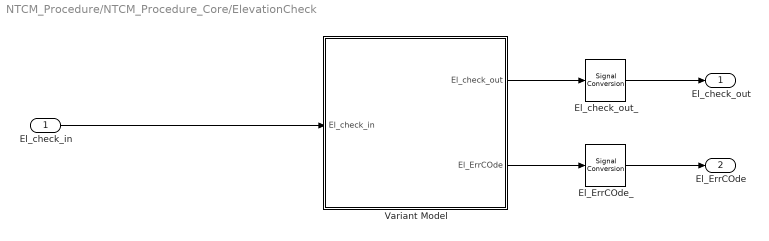
== system NTCM_Procedure/NTCM_Procedure_Core/ElevationCheck ==
  El_check_in : Inport
  El_ErrCOde_ : SignalConversion  OverrideOpt=off
  El_check_out_ : SignalConversion  OverrideOpt=off
  Variant Model : Subsystem  Variant=on  VariantActivationTime=code compile
  El_check_out : Outport
  El_ErrCOde : Outport  Port=2
  wires:
  El_check_in/1 -> Variant Model/1(El_check_in)
  Variant Model/2(El_ErrCOde) -> El_ErrCOde_/1
  Variant Model/1(El_check_out) -> El_check_out_/1
  El_check_out_/1 -> El_check_out/1
  El_ErrCOde_/1 -> El_ErrCOde/1

== system NTCM_Procedure/NTCM_Procedure_Core/LocalTime ==
  IppPosRad : Inport
  UTC : Inport  Port=2
  LocalTime : MATLAB Function  RTWFcnName=Local_time
      settings: RTWFileNameOpts=Use function name
  LT : Outport
  wires:
  UTC/1 -> LocalTime/2(UTC)
  LocalTime/1(LT) -> LT/1
  IppPosRad/1 -> LocalTime/1(IppPosRad)

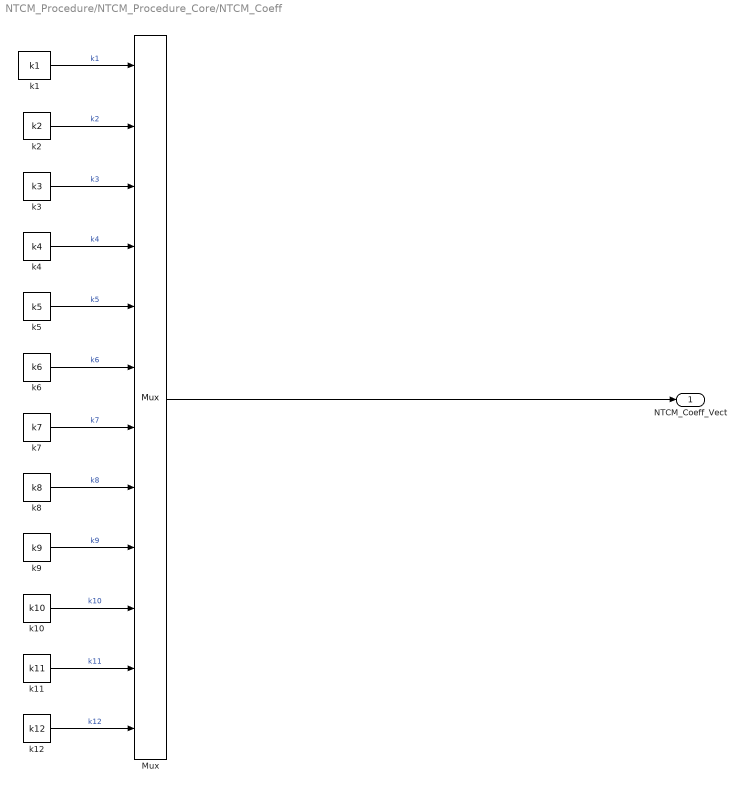
== system NTCM_Procedure/NTCM_Procedure_Core/NTCM_Coeff ==
  Mux : Mux  Inputs=12
  k1 : Constant  Value=k1
  k10 : Constant  Value=k10
  k11 : Constant  Value=k11
  k12 : Constant  Value=k12
  k2 : Constant  Value=k2
  k3 : Constant  Value=k3
  k4 : Constant  Value=k4
  k5 : Constant  Value=k5  VectorParams1D=off
  k6 : Constant  Value=k6
  k7 : Constant  Value=k7
  k8 : Constant  Value=k8
  k9 : Constant  Value=k9
  NTCM_Coeff_Vect : Outport  PortDimensions=[12,1]
  wires:
  k1/1 -> Mux/1  "k1"
  k2/1 -> Mux/2  "k2"
  k3/1 -> Mux/3  "k3"
  k4/1 -> Mux/4  "k4"
  k5/1 -> Mux/5  "k5"
  k6/1 -> Mux/6  "k6"
  k7/1 -> Mux/7  "k7"
  k8/1 -> Mux/8  "k8"
  k9/1 -> Mux/9  "k9"
  k10/1 -> Mux/10  "k10"
  k11/1 -> Mux/11  "k11"
  k12/1 -> Mux/12  "k12"
  Mux/1 -> NTCM_Coeff_Vect/1

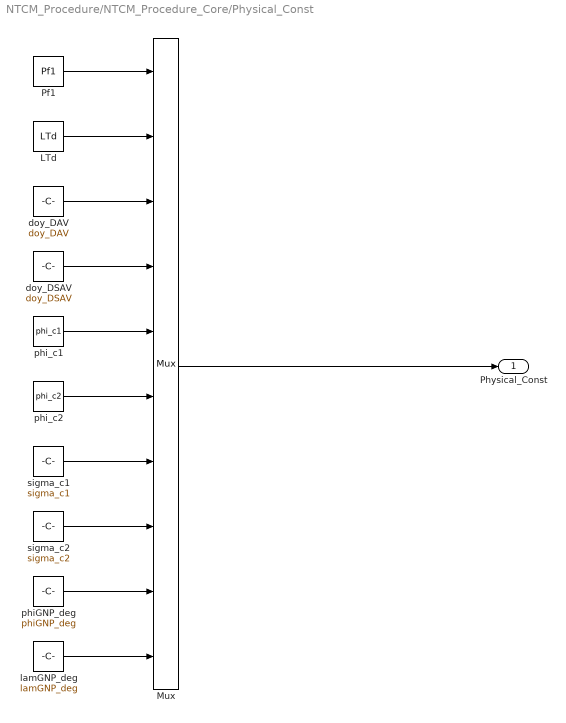
== system NTCM_Procedure/NTCM_Procedure_Core/Physical_Const ==
  LTd : Constant  Value=LTd
  Mux : Mux  Inputs=10
  Pf1 : Constant  Value=Pf1
  doy_DAV : Constant  Value=doy_DAV
  doy_DSAV : Constant  Value=doy_DSAV
  lamGNP_deg : Constant  Value=lamGNP_deg
  phiGNP_deg : Constant  Value=phiGNP_deg
  phi_c1 : Constant  Value=phi_c1
  phi_c2 : Constant  Value=phi_c2
  sigma_c1 : Constant  Value=sigma_c1
  sigma_c2 : Constant  Value=sigma_c2
  Physical_Const : Outport  PortDimensions=[10,1]
  wires:
  Pf1/1 -> Mux/1
  LTd/1 -> Mux/2
  doy_DAV/1 -> Mux/3
  doy_DSAV/1 -> Mux/4
  phi_c1/1 -> Mux/5
  phi_c2/1 -> Mux/6
  sigma_c1/1 -> Mux/7
  sigma_c2/1 -> Mux/8
  phiGNP_deg/1 -> Mux/9
  lamGNP_deg/1 -> Mux/10
  Mux/1 -> Physical_Const/1

== system NTCM_Procedure/ErrorMnG/Variant Subsystem/ErrorMnG  ==
  ErrorCodeCheckOut : Inport
  ErrorCodeCore : Inport  Port=2
  ErrorCodeCheckIn : Inport  Port=3
  Mux : Mux  Inputs=3
  ErrorCode : Outport
  wires:
  Mux/1 -> ErrorCode/1
  ErrorCodeCore/1 -> Mux/2
  ErrorCodeCheckOut/1 -> Mux/1
  ErrorCodeCheckIn/1 -> Mux/3

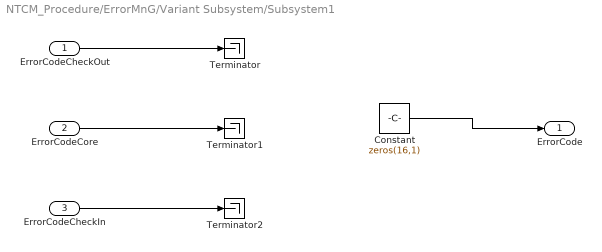
== system NTCM_Procedure/ErrorMnG/Variant Subsystem/Subsystem1 ==
  ErrorCodeCheckOut : Inport
  ErrorCodeCore : Inport  Port=2
  ErrorCodeCheckIn : Inport  Port=3
  Constant : Constant  Value=zeros(16,1)  OutDataTypeStr=uint16
  Terminator : Terminator
  Terminator1 : Terminator
  Terminator2 : Terminator
  ErrorCode : Outport
  wires:
  ErrorCodeCheckOut/1 -> Terminator/1
  ErrorCodeCore/1 -> Terminator1/1
  ErrorCodeCheckIn/1 -> Terminator2/1
  Constant/1 -> ErrorCode/1

== system NTCM_Procedure/NTCM_Procedure_Core/ElevationCheck/Variant Model ==
  note: 1) Add Subsystem or Model blocks as valid variant choices.
      | 2) You cannot connect blocks at this level. At simulation, connectivity is automatically
      | determined, based on the active variant and port name matching.
  El_check_in : Inport
  ElevationCheck : Subsystem  Description=|  TreatAsAtomicUnit=on  RTWFcnName=ElevCheck  VariantControl=CheckFlag  ReferencedSubsystem=ElevationCheck
      | # Test Point
      |  FUNCTION:
      |  ------
      |  Positivity elevetaion check 
      | 
      |  INPUT:
      |  ------
      |  El_check_in=> Satellite Elevation [rad]
      | 
      |  OUTPUT:
      | ------
      |  El_check_out=> Limited Elevation 
      |  El_ErrCOde => Elevation out of range error code
      settings: RTWFcnNameOpts=User specified  RTWFileNameOpts=Use function name
  ElevationCheck_ByPass : Subsystem  TreatAsAtomicUnit=on  VariantControl=(default)  ReferencedSubsystem=ElevationCheck_ByPass
  El_check_out : Outport
  El_ErrCOde : Outport  Port=2

== matlab function NTCM_Procedure/NTCM_Procedure_Core/Deg2Radllh1 ==
  settings: description=|
      | *Compute_Sun
      | *
      | *
      | *
      | *
      | *
      | *
      | *
  data: llhDeg input; llhRad output
function llhRad  = Deg2Radllh(llhDeg)
llhRad=llhDeg;
llhRad(1,1)=deg2rad(llhRad(1,1));
llhRad(2,1)=deg2rad(llhRad(2,1));

end

== matlab function NTCM_Procedure/NTCM_Procedure_Core/Deg2Radllh2 ==
  settings: description=|
      | *Compute_Sun
      | *
      | *
      | *
      | *
      | *
      | *
      | *
  data: llhDeg input; llhRad output
function llhRad  = Deg2Radllh(llhDeg)
llhRad=llhDeg;
llhRad(1,1)=deg2rad(llhRad(1,1));
llhRad(2,1)=deg2rad(llhRad(2,1));

end

== matlab function NTCM_Procedure/NTCM_Procedure_Core/LocalTime/LocalTime ==
  data: IppPosRad input; LT output; UTC input
function LT = fcn(IppPosRad,UTC)
% Compute Time Zone
LT=0;
timeZone   = -(IppPosRad(2,1)*180/pi/15);
% apply local time-zone
LT = (UTC - timeZone);

== matlab function NTCM_Procedure/NTCM_Procedure_Core/Compute_sTEC/Mapping_fun ==
  data: sTEC output; vTEC input; ele_rad input
function sTEC=Mapping_fun(vTEC,ele_rad)
% Mapping Function using: R=6371Km and H=450Km 
sTEC=0;
MF = 1./ sqrt(1-(0.934027268728925.*sin(0.9782*(pi/2-ele_rad))).^2);                             % ******  Eq.33
sTEC = vTEC .* MF;                                                                           % ******  Eq.16

== matlab function NTCM_Procedure/NTCM_Procedure_Core/Compute_IonoDelay/Compute_Delay ==
  data: delay_m output; sTEC input; fCarr input
function delay_m= Compute_Delay(sTEC,fCarr)
% Compute Ionospheric Delay according to signal carrier frequency 
delay_m=0;
b = cast(round(fCarr),"uint32");
if (b==0)
        delay_m = 0;
else
        delay_m = sTEC .*(40.3.*1e16)./fCarr.^2;                                                      % ******  Eq.1

end
end
